simulink model "Sensors_s"  (R2023a)
settings: Solver=VariableStepAuto  StartTime=0.0  StopTime=10.0  RelTol=1e-3
undefined symbols (not defined in the file): noise_seed_a_y, noise_seed_gamma, noise_seed_T_s, noise_seed_theta1, noise_seed_theta2_dot, noise_seed_v, noise_var_a_y, noise_var_gamma, noise_var_T_s, noise_var_theta1, noise_var_theta2_dot, noise_var_v, sens_Tupd_a_y, sens_Tupd_gamma, sens_Tupd_T_s, sens_Tupd_theta1, sens_Tupd_theta2_dot, sens_Tupd_v, sensors_on
settings Model: Creator=Tan_Tram  LastModifiedBy=Tan_Tram

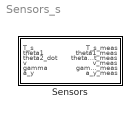
== system Sensors_s ==
  Sensors : Subsystem

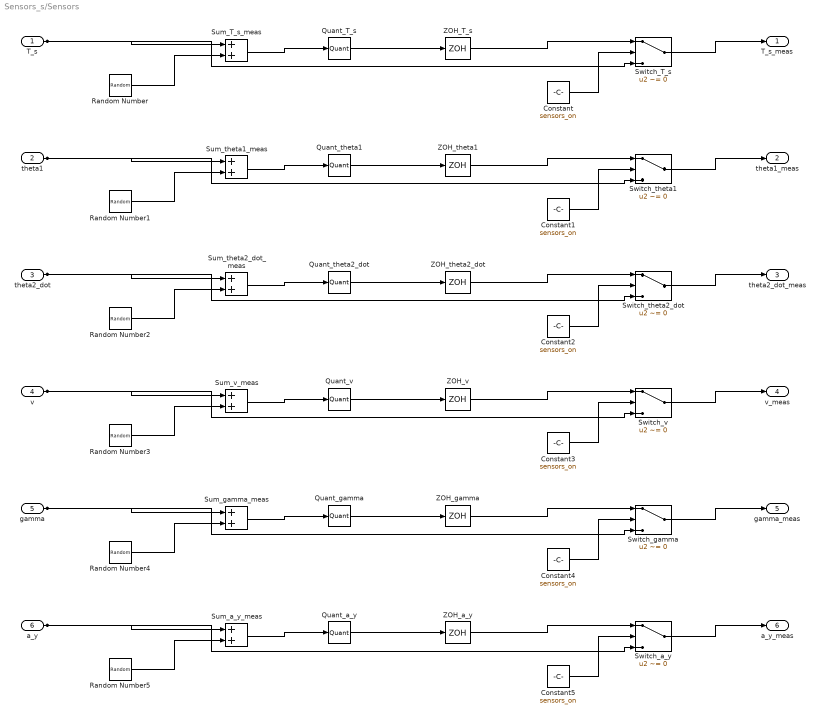
== system Sensors_s/Sensors ==
  T_s : Inport
  theta1 : Inport  Port=2
  theta2_dot : Inport  Port=3
  v : Inport  Port=4
  gamma : Inport  Port=5
  a_y : Inport  Port=6
  Constant{,1..5} (6 alike) : Constant  Value=sensors_on
  Quant_T_s : Quantizer  QuantizationInterval=sens_delta_T_s
  Quant_a_y : Quantizer  QuantizationInterval=sens_delta_a_y
  Quant_gamma : Quantizer  QuantizationInterval=sens_delta_gamma
  Quant_theta1 : Quantizer  QuantizationInterval=sens_delta_theta1
  Quant_theta2_dot : Quantizer  QuantizationInterval=sens_delta_theta2_dot
  Quant_v : Quantizer  QuantizationInterval=sens_delta_v
  Random Number : RandomNumber  Variance=noise_var_T_s  Seed=noise_seed_T_s  SampleTime=sens_Tupd_T_s
  Random Number1 : RandomNumber  Variance=noise_var_theta1  Seed=noise_seed_theta1  SampleTime=sens_Tupd_theta1
  Random Number2 : RandomNumber  Variance=noise_var_theta2_dot  Seed=noise_seed_theta2_dot  SampleTime=sens_Tupd_theta2_dot
  Random Number3 : RandomNumber  Variance=noise_var_v  Seed=noise_seed_v  SampleTime=sens_Tupd_v
  Random Number4 : RandomNumber  Variance=noise_var_gamma  Seed=noise_seed_gamma  SampleTime=sens_Tupd_gamma
  Random Number5 : RandomNumber  Variance=noise_var_a_y  Seed=noise_seed_a_y  SampleTime=sens_Tupd_a_y
  Sum_T_s_meas : Sum
  Sum_a_y_meas : Sum
  Sum_gamma_meas : Sum
  Sum_theta1_meas : Sum
  Sum_theta2_dot_meas : Sum
  Sum_v_meas : Sum
  Switch_T_s : Switch  Criteria=u2 ~= 0  SaturateOnIntegerOverflow=off  InputSameDT=off
  Switch_a_y : Switch  Criteria=u2 ~= 0  SaturateOnIntegerOverflow=off  InputSameDT=off
  Switch_gamma : Switch  Criteria=u2 ~= 0  SaturateOnIntegerOverflow=off  InputSameDT=off
  Switch_theta1 : Switch  Criteria=u2 ~= 0  SaturateOnIntegerOverflow=off  InputSameDT=off
  Switch_theta2_dot : Switch  Criteria=u2 ~= 0  SaturateOnIntegerOverflow=off  InputSameDT=off
  Switch_v : Switch  Criteria=u2 ~= 0  SaturateOnIntegerOverflow=off  InputSameDT=off
  ZOH_T_s : ZeroOrderHold  SampleTime=sens_Tupd_T_s
  ZOH_a_y : ZeroOrderHold  SampleTime=sens_Tupd_a_y
  ZOH_gamma : ZeroOrderHold  SampleTime=sens_Tupd_gamma
  ZOH_theta1 : ZeroOrderHold  SampleTime=sens_Tupd_theta1
  ZOH_theta2_dot : ZeroOrderHold  SampleTime=sens_Tupd_theta2_dot
  ZOH_v : ZeroOrderHold  SampleTime=sens_Tupd_v
  T_s_meas : Outport
  theta1_meas : Outport  Port=2
  theta2_dot_meas : Outport  Port=3
  v_meas : Outport  Port=4
  gamma_meas : Outport  Port=5
  a_y_meas : Outport  Port=6
  wires:
  T_s/1 -> Sum_T_s_meas/1, Switch_T_s/3
  Random Number/1 -> Sum_T_s_meas/2
  Sum_T_s_meas/1 -> Quant_T_s/1
  Quant_T_s/1 -> ZOH_T_s/1
  ZOH_T_s/1 -> Switch_T_s/1
  Constant/1 -> Switch_T_s/2
  Switch_T_s/1 -> T_s_meas/1
  theta1/1 -> Sum_theta1_meas/1, Switch_theta1/3
  Random Number1/1 -> Sum_theta1_meas/2
  Sum_theta1_meas/1 -> Quant_theta1/1
  Quant_theta1/1 -> ZOH_theta1/1
  ZOH_theta1/1 -> Switch_theta1/1
  Constant1/1 -> Switch_theta1/2
  Switch_theta1/1 -> theta1_meas/1
  theta2_dot/1 -> Sum_theta2_dot_meas/1, Switch_theta2_dot/3
  Random Number2/1 -> Sum_theta2_dot_meas/2
  Sum_theta2_dot_meas/1 -> Quant_theta2_dot/1
  Quant_theta2_dot/1 -> ZOH_theta2_dot/1
  ZOH_theta2_dot/1 -> Switch_theta2_dot/1
  Constant2/1 -> Switch_theta2_dot/2
  Switch_theta2_dot/1 -> theta2_dot_meas/1
  v/1 -> Sum_v_meas/1, Switch_v/3
  Random Number3/1 -> Sum_v_meas/2
  Sum_v_meas/1 -> Quant_v/1
  Quant_v/1 -> ZOH_v/1
  ZOH_v/1 -> Switch_v/1
  Constant3/1 -> Switch_v/2
  Switch_v/1 -> v_meas/1
  gamma/1 -> Sum_gamma_meas/1, Switch_gamma/3
  Random Number4/1 -> Sum_gamma_meas/2
  Sum_gamma_meas/1 -> Quant_gamma/1
  Quant_gamma/1 -> ZOH_gamma/1
  ZOH_gamma/1 -> Switch_gamma/1
  Constant4/1 -> Switch_gamma/2
  Switch_gamma/1 -> gamma_meas/1
  a_y/1 -> Sum_a_y_meas/1, Switch_a_y/3
  Random Number5/1 -> Sum_a_y_meas/2
  Sum_a_y_meas/1 -> Quant_a_y/1
  Quant_a_y/1 -> ZOH_a_y/1
  ZOH_a_y/1 -> Switch_a_y/1
  Constant5/1 -> Switch_a_y/2
  Switch_a_y/1 -> a_y_meas/1
